simulink model "pendulum_openloop_anim_WIP"  (Simulink 9.2)
settings: Solver=ode45  StartTime=0.0  StopTime=inf  RelTol=1e-3  EnableMultiTasking=on
values from neighbouring files (symbols this model uses):
  g = 9.81    [pendulum_sys_init_NOsolution.m]    (also in pendulum_sys_init_WIP.m)
  kc = 2    [pendulum_sys_init_NOsolution.m]    (also in pendulum_sys_init_WIP.m)
  ke = 2    [pendulum_sys_init_NOsolution.m]    (also in pendulum_sys_init_WIP.m)
  Ktilde = place(Atilde, Btilde, P)    [pendulum_sys_init_WIP.m]
  l = 1    [pendulum_sys_init_NOsolution.m]    (also in pendulum_sys_init_WIP.m = 1.5)
  M = 10    [pendulum_sys_init_NOsolution.m]    (also in pendulum_sys_init_WIP.m)
  m = 2    [pendulum_sys_init_NOsolution.m]    (also in pendulum_sys_init_WIP.m = 0.5)
  ra = 10    [pendulum_sys_init_NOsolution.m]    (also in pendulum_sys_init_WIP.m)
  rr = .1    (= 0.1)    [pendulum_sys_init_NOsolution.m]    (also in pendulum_sys_init_WIP.m)
undefined symbols (not defined in the file or in its folder): pendolo_sys_diff
libraries: vrlib x1
settings Model: Creator=Titano  LastModifiedBy=Varazslav
settings OptimizationCC: BlockReduction=off  DefaultParameterBehavior=Inlined  BufferReuse=off  ExpressionDepthLimit=2147483647  InitFltsAndDblsToZero=on
settings DebuggingCC: SolverPrmCheckMsg=warning
settings SimscapeCC: SimscapeNormalizeSystem=off
settings SimMechanicsCC: VisDuringSimulation=on
settings ConfigurationSet: Description=SimMechanics 2G

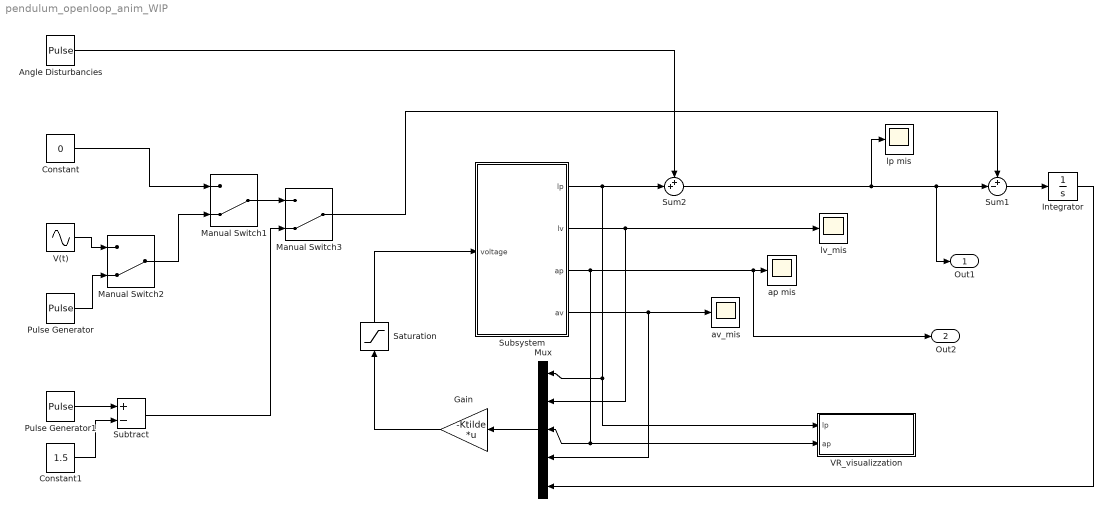
== system pendulum_openloop_anim_WIP ==
  Angle Disturbancies : DiscretePulseGenerator  PulseType=Time based  Period=5  PulseWidth=10
  Constant : Constant  Value=0
  Constant1 : Constant  Value=1.5
  Gain : Gain  Gain=-Ktilde  Multiplication=Matrix(K*u)
  Integrator : Integrator
  Manual Switch1 : ManualSwitch  CurrentSetting=0
  Manual Switch2 : ManualSwitch  CurrentSetting=0
  Manual Switch3 : ManualSwitch  CurrentSetting=0
  Mux : Mux  Inputs=5
  Pulse Generator : DiscretePulseGenerator  PulseType=Time based  Period=20  PulseWidth=50
  Pulse Generator1 : DiscretePulseGenerator  PulseType=Time based  Amplitude=3  Period=20  PulseWidth=50
  Saturation : Saturate  UpperLimit=24  LowerLimit=-24
  Subsystem : Subsystem
  Subtract : Sum  Inputs=+-
  Sum1 : Sum  Inputs=+-|
  Sum2 : Sum  Inputs=++|
  "V(t) " : Sin  Amplitude=2  Frequency=0.8  SampleTime=0
  VR_visualizzation : Subsystem
  ap mis : Scope
  "av_mis " : Scope
  lp mis : Scope
  lv_mis : Scope
  Out1 : Outport
  Out2 : Outport  Port=2
  wires:
  Gain/1 -> Saturation/1
  Subsystem/2(lv) -> Mux/2, lv_mis/1
  Subsystem/4(av) -> Mux/4, "av_mis "/1
  Mux/1 -> Gain/1
  Integrator/1 -> Mux/5
  Sum1/1 -> Integrator/1
  Constant/1 -> Manual Switch1/1
  Manual Switch1/1 -> Manual Switch3/1
  Saturation/1 -> Subsystem/1(voltage)
  Subsystem/1(lp) -> Sum2/2, Mux/1, VR_visualizzation/1(lp)
  Angle Disturbancies/1 -> Sum2/1
  "V(t) "/1 -> Manual Switch2/1
  Pulse Generator/1 -> Manual Switch2/2
  Manual Switch2/1 -> Manual Switch1/2
  Subsystem/3(ap) -> Out2/1, ap mis/1, Mux/3, VR_visualizzation/2(ap)
  Sum2/1 -> lp mis/1, Out1/1, Sum1/2
  Manual Switch3/1 -> Sum1/1
  Constant1/1 -> Subtract/2
  Pulse Generator1/1 -> Subtract/1
  Subtract/1 -> Manual Switch3/2

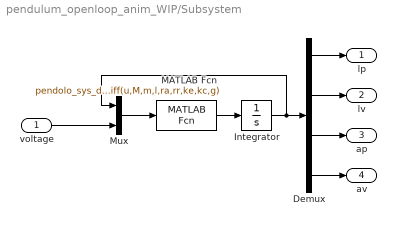
== system pendulum_openloop_anim_WIP/Subsystem ==
  voltage : Inport
  Demux : Demux
  Integrator : Integrator  InitialCondition=[0 0.0 0.15 0]
  MATLAB Fcn : MATLABFcn  MATLABFcn=pendolo_sys_diff(u,M,m,l,ra,rr,ke,kc,g)
  Mux : Mux  Inputs=2
  lp : Outport
  lv : Outport  Port=2
  ap : Outport  Port=3
  av : Outport  Port=4
  wires:
  MATLAB Fcn/1 -> Integrator/1
  Integrator/1 -> Demux/1, Mux/1
  Demux/4 -> av/1
  Demux/3 -> ap/1
  Demux/2 -> lv/1
  Demux/1 -> lp/1
  Mux/1 -> MATLAB Fcn/1
  voltage/1 -> Mux/2

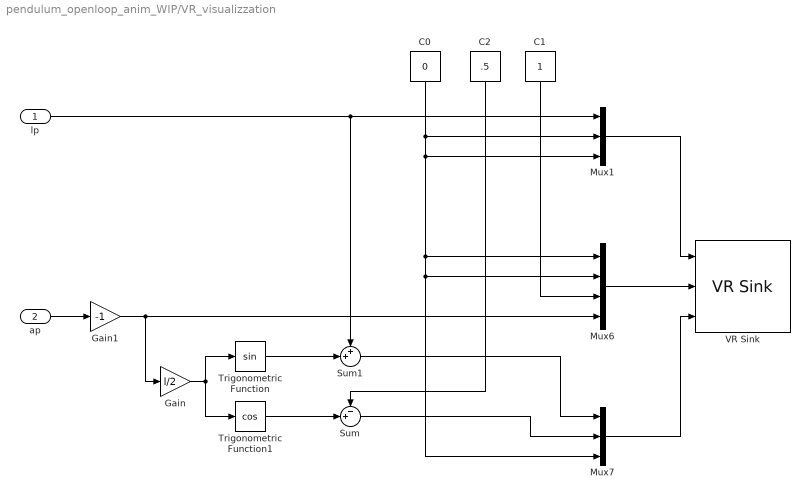
== system pendulum_openloop_anim_WIP/VR_visualizzation ==
  lp : Inport
  ap : Inport  Port=2
  C0 : Constant  Value=0
  C1 : Constant
  C2 : Constant  Value=.5
  Gain : Gain  Gain=l/2
  Gain1 : Gain  Gain=-1
  Mux1 : Mux  Inputs=3
  Mux6 : Mux
  Mux7 : Mux  Inputs=3
  Sum : Sum  Inputs=-+|
  Sum1 : Sum  Inputs=++|
  Trigonometric Function : Trigonometry
  Trigonometric Function1 : Trigonometry  Operator=cos
  VR Sink : vrlib/VR Sink  InstantiateOnLoad=on  SampleTime=0.02  ViewEnable=on  RemoteChange=off  RemoteView=off  FieldsWritten=carrello.translation.3.1.double#asta.rotation.4.1.double#asta.translation.3.1.double  WorldFileName=vrml1.wrl  AutoView=on  VideoDimensions=[]  AllowVariableSize=off  FigureProperties="{'Position', 'Name', 'Viewpoint', 'CameraBound', 'CameraDirection', 'CameraPosition', 'CameraUpVector', 'ZoomFactor', 'Antialiasing', 'Headlight', 'Lighting', 'NavPanel', 'Sound', 'StatusBar', 'Stereo3D', 'Stereo3DCameraOffset', 'Stereo3DHIT', 'ToolBar', 'Textures', 'Transparency', 'Triad', 'Wireframe', 'NavZones', 'NavMode', 'NavSpeed', 'CaptureFileFormat', 'CaptureFileName', 'Record2DCompressMethod', 'Record2DCompressQuality', 'Record2D', 'Record2DFileName', 'Record2DFPS'; [7.8200000000000000e+02   2.4800000000000000e+02   5.7600000000000000e+02   3.5000000000000000e+02], '', '', 'on', [0.0000000000000000e+00   0.0000000000000000e+00  -1.0000000000000000e+00], [0.0000000000000000e+00   0.0000000000000000e+00   3.0000000000000000e+00], [0.0000000000000000e+00   1.0000000000000000e+00   0.0000000000000000e+00], [1.0000000000000000e+00], 'on', 'on', 'on', 'halfbar', 'on', 'on', 'off', [1.0000000149011612e-01], [0.0000000000000000e+00], 'on', 'on', 'on', 'none', 'off', 'off', 'walk', 'normal', 'tif', '%f_anim_%n.tif', 'auto', [7.5000000000000000e+01], 'off', '%f_anim_%n.avi', 'auto'}"
      settings: SourceProductBaseCode=VR
  wires:
  Mux1/1 -> VR Sink/1
  Mux7/1 -> VR Sink/3
  lp/1 -> Mux1/1, Sum1/1
  C0/1 -> Mux1/2, Mux1/3, Mux6/1, Mux6/2, Mux7/3
  ap/1 -> Gain1/1
  C1/1 -> Mux6/3
  Trigonometric Function/1 -> Sum1/2
  Trigonometric Function1/1 -> Sum/2
  Sum1/1 -> Mux7/1
  Sum/1 -> Mux7/2
  C2/1 -> Sum/1
  Gain/1 -> Trigonometric Function/1, Trigonometric Function1/1
  Gain1/1 -> Mux6/4, Gain/1
  Mux6/1 -> VR Sink/2
